simulink model "NCS_Simulation"  (R2019a)
settings: Solver=ode4  StartTime=0.0  StopTime=200  FixedStep=0.004  MaxStep=0.01  RelTol=1e-3
values from neighbouring files (symbols this model uses):
  CAN2EthernetDelay = 0.000    (= 0)    [Parameter.m]
  CycleTime_Sensor = 1/1000    (= 0.001)    [Parameter.m]
  Ethernet2CANDelay = 0.005    [Parameter.m]
  n = 0.001    [Parameter.m]
  nW_ges = 8    [Parameter.m]
  ReferenceDelay = 0.0    (= 0)    [Parameter.m]
undefined symbols (not defined in the file or in its folder): BUSCapacity, controlGate, entity, m, ReadData, ReadSize, v0
libraries: NCS_Library x250, simulink x12
(part 3 of 3)

== system NCS_Simulation/Network/Ethernet (Ring) CAN/Consist 1/Fieldbus 1/Gateway1/CAN Interface/Save Data ==
  Type : Inport
  Data : Inport  Port=2
  FLUSH : Inport  Port=3
  Add : Sum
  Delay : Delay  DelayLength=1  InitialCondition=1
  Detect Change : simulink/Logic and Bit Operations/Detect Change  vinit=0  OutDataTypeStr=boolean
  Detect Change1 : simulink/Logic and Bit Operations/Detect Change  vinit=0  OutDataTypeStr=boolean
  Display : Display
  Display1 : Display
  Display2 : Display
  Hold Data : Stateflow chart  TreatAsAtomicUnit=on
  MATLAB Function : MATLAB Function  TreatAsAtomicUnit=on
  Memory : Memory  InheritSampleTime=on
  OutData : Outport
  wires:
  Hold Data/1(OutData) -> Display/1, OutData/1
  Delay/1 -> MATLAB Function/1(refresh)
  Data/1 -> Detect Change1/1, MATLAB Function/4(Data), Display1/1
  Type/1 -> Detect Change/1, MATLAB Function/3(Type), Display2/1
  MATLAB Function/1(M_Data) -> Memory/1, Hold Data/2(InData)
  FLUSH/1 -> Delay/1, Hold Data/1(Flush)
  Memory/1 -> MATLAB Function/5(M_Data_old)
  Add/1 -> MATLAB Function/2(write)
  Detect Change/1 -> Add/1
  Detect Change1/1 -> Add/2

== system NCS_Simulation/Network/Ethernet (Ring) CAN/Consist 1/Fieldbus 1/Gateway1/Ethernet Interface/Enabled Subsystem ==
  In1 : Inport
  Enable : EnablePort
  Out1 : Outport
  wires:
  In1/1 -> Out1/1

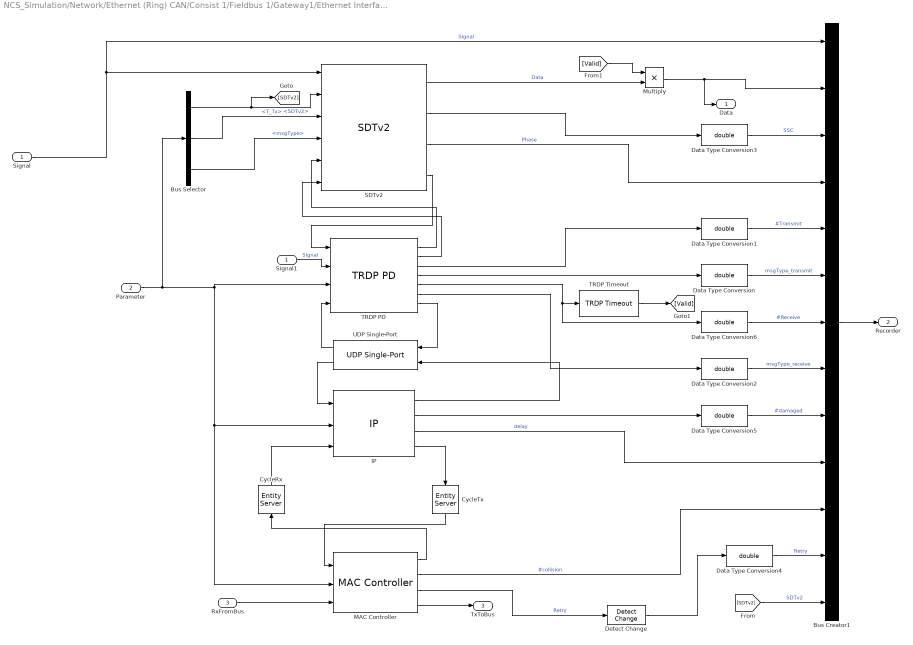
== system NCS_Simulation/Network/Ethernet (Ring) CAN/Consist 1/Fieldbus 1/Gateway1/Ethernet Interface/Protocol Stack ==
  Signal : Inport
  Parameter : Inport  Port=2
  RxFromBus : Inport  Port=3
  Bus Creator1 : BusCreator  Inputs=13
  Bus Selector : BusSelector  OutputSignals=SDTv2,T_Tx,msgType
  CycleRx : EntityServer  InputPortMessageModes=m  OutputPortMessageModes=m  Capacity=inf  ServiceTimeValue=CycleRx
  CycleTx : EntityServer  InputPortMessageModes=m  OutputPortMessageModes=m  Capacity=inf  ServiceTimeValue=CycleTx
  Data Type Conversion{,1..6} (7 alike) : DataTypeConversion  OutDataTypeStr=double
  Detect Change : simulink/Logic and Bit Operations/Detect Change  vinit=0  OutDataTypeStr=boolean
  IP : NCS_Library/Network/ETB/OSI Layers/IP  SystemSampleTime=-1
  MAC Controller : NCS_Library/Network/ETB/OSI Layers/MAC Controller  SystemSampleTime=-1
  Multiply : Product
  SDTv2 : NCS_Library/Network/ETB/OSI Layers/SDTv2  SystemSampleTime=-1
  Signal1 : InportShadow
  TRDP PD : NCS_Library/Network/ETB/OSI Layers/TRDP PD  SystemSampleTime=-1
  TRDP Timeout : NCS_Library/Network/ETB/OSI Layers/TRDP Timeout  SystemSampleTime=-1
  UDP Single-Port : NCS_Library/Network/ETB/OSI Layers/UDP Single-Port  SystemSampleTime=-1
  Data : Outport
  Recorder : Outport  Port=2
  TxToBus : Outport  Port=3
  wires:
  TRDP Timeout/1 -> [Valid]
  [Valid] -> Multiply/1
  SDTv2/1 -> Multiply/2  "Data"
  Multiply/1 -> Bus Creator1/2, Data/1
  Signal1/1 -> TRDP PD/2  "Signal"
  CycleTx/1 -> MAC Controller/1
  IP/4 -> CycleTx/1
  MAC Controller/1 -> CycleRx/1
  CycleRx/1 -> IP/3
  IP/3 -> Bus Creator1/10  "delay"
  IP/2 -> Data Type Conversion5/1
  TRDP PD/6 -> Data Type Conversion2/1
  TRDP PD/5 -> Data Type Conversion6/1, TRDP Timeout/1
  TRDP PD/4 -> Data Type Conversion/1
  TRDP PD/3 -> Data Type Conversion1/1
  SDTv2/3 -> Bus Creator1/4  "Phase"
  SDTv2/2 -> Data Type Conversion3/1
  [SDTv2] -> Bus Creator1/13  "SDTv2"
  RxFromBus/1 -> MAC Controller/3
  UDP Single-Port/2 -> IP/1
  IP/1 -> UDP Single-Port/2
  UDP Single-Port/1 -> TRDP PD/4
  MAC Controller/2 -> Bus Creator1/11  "#collision"
  Signal/1 -> Bus Creator1/1, SDTv2/1  "Signal"
  Parameter/1 -> Bus Selector/1, IP/2, MAC Controller/2, TRDP PD/3
  Data Type Conversion/1 -> Bus Creator1/6  "msgType_transmit"
  Bus Creator1/1 -> Recorder/1
  TRDP PD/7 -> UDP Single-Port/1
  SDTv2/4 -> TRDP PD/1
  TRDP PD/2 -> SDTv2/6
  Bus Selector/2 -> SDTv2/3  "<T_Tx>"
  TRDP PD/1 -> SDTv2/5
  Bus Selector/3 -> SDTv2/4  "<msgType>"
  MAC Controller/4 -> TxToBus/1
  MAC Controller/3 -> Detect Change/1  "Retry"
  Detect Change/1 -> Data Type Conversion4/1
  Bus Selector/1 -> [SDTv2], SDTv2/2  "<SDTv2>"
  Data Type Conversion1/1 -> Bus Creator1/5  "#Transmit"
  Data Type Conversion2/1 -> Bus Creator1/8  "msgType_receive"
  Data Type Conversion3/1 -> Bus Creator1/3  "SSC"
  Data Type Conversion4/1 -> Bus Creator1/12  "Retry"
  Data Type Conversion5/1 -> Bus Creator1/9  "#damaged"
  Data Type Conversion6/1 -> Bus Creator1/7  "#Receive"

== system NCS_Simulation/Network/Ethernet (Ring) CAN/Consist 1/Fieldbus 1/Gateway1/Ethernet Interface/Subsystem4 ==
  Data : Inport
  Add3 : Sum  Inputs=-+-+
  Chart : Stateflow chart  TreatAsAtomicUnit=on
  Clock : Clock
  Compare To Zero1 : simulink/Logic and Bit Operations/Compare To Zero  relop=>=  OutDataTypeStr=uint8
  Constant8 : Constant  Value=T_Tx_CAN
  Constant9 : Constant  Value=1e-10
  Detect Change : simulink/Logic and Bit Operations/Detect Change  vinit=0  OutDataTypeStr=boolean
  Display : Display
  Display1 : Display
  Display2 : Display
  MATLAB Function : MATLAB Function  TreatAsAtomicUnit=on
  Memory1 : Memory  InheritSampleTime=on
  Multiply1 : Product
  Save num release : Subsystem
  Push : Outport
  wires:
  MATLAB Function/1(NEW) -> Display/1, Chart/2(NEW)
  Detect Change/1 -> MATLAB Function/2(Change)
  Compare To Zero1/1 -> Chart/1(TIME), Display1/1, Save num release/Enable
  Chart/1(Push) -> Push/1
  Data/1 -> MATLAB Function/1(Data), Detect Change/1, Display2/1
  Clock/1 -> Add3/2
  Multiply1/1 -> Add3/1
  Memory1/1 -> Multiply1/1, Save num release/1(Time)
  Constant8/1 -> Add3/3, Multiply1/2  "T_Tx"
  Save num release/1(Out1) -> Memory1/1
  Constant9/1 -> Add3/4  "Compensate numeric drift"
  Add3/1 -> Compare To Zero1/1

== system NCS_Simulation/Network/Ethernet (Ring) CAN/Consist 1/Fieldbus 1/Gateway1/Ethernet Interface/User Interface ==
  note: User defined Parameters
  Add : Sum  Inputs=+-
  Bus Creator : BusCreator  Inputs=8
  Constant : Constant  Value=Address  OutDataTypeStr=uint16
  Constant1 : Constant  Value=Destination  OutDataTypeStr=uint16
  Constant2 : Constant  Value=0  OutDataTypeStr=double
  Constant3 : Constant  Value=3  OutDataTypeStr=uint8
  Constant4 : Constant  Value=SDTv2  OutDataTypeStr=double
  Constant5 : Constant
  Constant6 : Constant  Value=Port  OutDataTypeStr=uint16
  Constant7 : Constant  Value=ReplyAddress  OutDataTypeStr=uint16
  MATLAB Function : MATLAB Function  TreatAsAtomicUnit=on
  MATLAB Function1 : MATLAB Function  TreatAsAtomicUnit=on
  Subscribe : Constant  Value=Subscribe  OutDataTypeStr=uint16
  Subsystem1 : Subsystem
  Subsystem2 : Subsystem
  Subsystem3 : Subsystem
  Out1 : Outport
  wires:
  Bus Creator/1 -> Out1/1
  Constant7/1 -> Subsystem3/1(In1)
  Constant5/1 -> Add/2
  Constant2/1 -> Bus Creator/6  "T_Tx"
  Constant1/1 -> Subsystem2/1(In1)
  Subsystem2/1(Out1) -> Bus Creator/2  "Destination"
  MATLAB Function/1(msgType) -> Bus Creator/7  "msgType"
  Subsystem3/1(Out1) -> Bus Creator/4  "ReplyAddress"
  Constant3/1 -> MATLAB Function/1(u)
  Subsystem1/1(Out1) -> Bus Creator/1  "Address"
  Constant/1 -> Subsystem1/1(In1)
  Constant4/1 -> Add/1
  MATLAB Function1/1(y) -> Bus Creator/3  "Subscribe"
  Constant6/1 -> Bus Creator/5  "Port"
  Subscribe/1 -> MATLAB Function1/1(u)
  Add/1 -> Bus Creator/8  "SDTv2"

== system NCS_Simulation/Network/Ethernet (Ring) CAN/Consist 1/Fieldbus 1/Gateway1/CAN Interface/CAN Interface/Re-Transmission Control ==
  IN : Inport
  ReTX : Inport  Port=2
  Reset : Inport  Port=3
  Discard Saved Message upon Success : EntityGate  InputPortMessageModes=m,m  OutputPortMessageModes=m  OperatingMode=Release gate
  Entity Sink : EntityTerminator  InputPortMessageModes=m  NumberEntitiesArrived=on
      settings: OutputPortMap=o0
  Re-Transmission Decision : EntityOutputSwitch  InputPortMessageModes=m  OutputPortMessageModes=m,m  SwitchAttributeName=Attribute1
  Re-transmit Saved Message upon Failure : EntityGate  InputPortMessageModes=m,m  OutputPortMessageModes=m  OperatingMode=Release gate
  OUT : Outport
  #TX : Outport  Port=2
  wires:
  Reset/1 -> Discard Saved Message upon Success/1
  ReTX/1 -> Re-transmit Saved Message upon Failure/1
  Entity Sink/1 -> #TX/1
  Discard Saved Message upon Success/1 -> Entity Sink/1
  Re-Transmission Decision/2 -> Discard Saved Message upon Success/2
  Re-transmit Saved Message upon Failure/1 -> OUT/1
  Re-Transmission Decision/1 -> Re-transmit Saved Message upon Failure/2
  IN/1 -> Re-Transmission Decision/1

== system NCS_Simulation/Network/Ethernet (Ring) CAN/Consist 1/Fieldbus 1/Gateway1/CAN Interface/CAN Interface/Reception Control/Compute ==
  rx_id : Inport  OutDataTypeStr=double  PortDimensions=1
  loss : Inport  Port=2  OutDataTypeStr=double  PortDimensions=1
  rx_rtr : Inport  Port=3  OutDataTypeStr=double  PortDimensions=1
  rx_data : Inport  Port=4  OutDataTypeStr=double  PortDimensions=1
  tx_id : Inport  Port=5  OutDataTypeStr=double  PortDimensions=1
  tx_rtr : Inport  Port=6  OutDataTypeStr=double  PortDimensions=1
  tx_data : Inport  Port=7  OutDataTypeStr=double  PortDimensions=1
  f : TriggerPort  TriggerType=function-call  VariantControl=Variant
      settings: CopyFcn=Stateflow.SLINSF.SimulinkMan.removeBlockPreDeleteFcn  PreDeleteFcn=Stateflow.SLINSF.SimulinkMan.unsafePredeleteFcn
  Lookup Table : Lookup  InputValues=IDRange  Table=2*ones(1,length(IDRange))-IDSubscription  LUTDesignUseExistingBP=off  LUTDesignAbsError=NaN
  MATLAB Function : MATLAB Function  TreatAsAtomicUnit=on
  Sum : Sum  Inputs=|++
  Status : Outport
  Ack : Outport  Port=2
  wires:
  tx_id/1 -> MATLAB Function/4(ID1)
  rx_rtr/1 -> MATLAB Function/2(RTR0)
  rx_id/1 -> MATLAB Function/1(ID0), Lookup Table/1
  Lookup Table/1 -> Sum/1
  loss/1 -> Sum/2, MATLAB Function/7(Loss)
  rx_data/1 -> MATLAB Function/3(Data0)
  tx_data/1 -> MATLAB Function/6(Data1)
  tx_rtr/1 -> MATLAB Function/5(RTR1)
  Sum/1 -> Status/1
  MATLAB Function/1(ACK) -> Ack/1

== system NCS_Simulation/Network/Ethernet (Ring) CAN/Consist 1/Fieldbus 1/Gateway1/CAN Interface/CAN Interface/Signal To CAN Message ==
  Data : Inport
  Entity Generator : EntityGenerator  OutputPortMessageModes=m  Period=T_Tx_CAN  GenerateEntityAtSimulationStart=off  GenerateAction=[entity.ID,entity.RTR,entity.Size,entity.f_St,entity.CommDelay,entity.Time, entity.SensorType] = initMessage();  AttributeName=ID|RTR|Size|Data|CommDelay|RndLoss  AttributeInitialValue=1|1|1|1|1|0  EntityType=Bus object  EntityTypeName=CAN_Message  EntityPriority=MsgID
  Set the Attributes of Messages : Subsystem  TreatAsAtomicUnit=on
  MsgOut : Outport
  wires:
  Data/1 -> Set the Attributes of Messages/1(InData)
  Entity Generator/1 -> MsgOut/1

== system NCS_Simulation/Network/Ethernet (Ring) CAN/Consist 1/Fieldbus 1/Gateway1/CAN Interface/CAN Interface/Simulink Function ==
  controlGate : TriggerPort  TriggerType=function-call  IsSimulinkFunction=on  FunctionName=controlGate  FunctionVisibility=scoped  VariantControl=Variant
  Message Send : MessageSend  OutputPortMessageModes=m
      settings: InputPortMap=u1
  u : ArgIn  DisableCoverage=on  ArgumentName=u
  ctrl : Outport
  wires:
  u/1 -> Message Send/1
  Message Send/1 -> ctrl/1

== system NCS_Simulation/Network/Ethernet (Ring) CAN/Consist 1/Fieldbus 1/Gateway1/CAN Interface/Entry Control/Enabled Subsystem ==
  Enable : EnablePort  StatesWhenEnabling=reset
  Constant : Constant
  Message Send3 : MessageSend  OutputPortMessageModes=m
      settings: InputPortMap=u1
  Out1 : Outport  OutputWhenDisabled=reset  InitialOutput=1
  wires:
  Message Send3/1 -> Out1/1
  Constant/1 -> Message Send3/1

== system NCS_Simulation/Network/Ethernet (Ring) CAN/Consist 1/Fieldbus 1/Gateway1/CAN Interface/Gate Control/Save last release time1 ==
  Time : Inport
  Enable : EnablePort
  Add : Sum
  Constant : Constant  OutDataTypeStr=uint32
  Data Type Conversion : DataTypeConversion  OutDataTypeStr=double
  Display : Display
  Out1 : Outport  InitialOutput=0
  wires:
  Time/1 -> Add/1
  Add/1 -> Data Type Conversion/1
  Constant/1 -> Add/2
  Data Type Conversion/1 -> Display/1, Out1/1

== system NCS_Simulation/Network/Ethernet (Ring) CAN/Consist 1/Fieldbus 1/Gateway1/Ethernet Interface/Subsystem4/Save num release ==
  Time : Inport
  Enable : EnablePort
  Add : Sum
  Constant : Constant  OutDataTypeStr=uint32
  Data Type Conversion : DataTypeConversion  OutDataTypeStr=double
  Display : Display
  Out1 : Outport  InitialOutput=0
  wires:
  Data Type Conversion/1 -> Out1/1, Display/1
  Constant/1 -> Add/2
  Add/1 -> Data Type Conversion/1
  Time/1 -> Add/1

== system NCS_Simulation/Network/Ethernet (Ring) CAN/Consist 1/Fieldbus 1/Gateway1/Ethernet Interface/User Interface/Subsystem1 ==
  In1 : Inport
  Constant : Constant  Value=0  OutDataTypeStr=uint16
  Constant1 : Constant  Value=0  OutDataTypeStr=uint16
  Mux : Mux  Inputs=3
  Out1 : Outport
  wires:
  Constant1/1 -> Mux/3
  Constant/1 -> Mux/2
  Mux/1 -> Out1/1
  In1/1 -> Mux/1

== system NCS_Simulation/Network/Ethernet (Ring) CAN/Consist 1/Fieldbus 1/Gateway1/Ethernet Interface/User Interface/Subsystem2 ==
  In1 : Inport
  Constant : Constant  Value=0  OutDataTypeStr=uint16
  Constant1 : Constant  Value=0  OutDataTypeStr=uint16
  Mux : Mux  Inputs=3
  Out1 : Outport
  wires:
  In1/1 -> Mux/1
  Mux/1 -> Out1/1
  Constant/1 -> Mux/2
  Constant1/1 -> Mux/3

== system NCS_Simulation/Network/Ethernet (Ring) CAN/Consist 1/Fieldbus 1/Gateway1/Ethernet Interface/User Interface/Subsystem3 ==
  In1 : Inport
  Constant : Constant  Value=0  OutDataTypeStr=uint16
  Constant1 : Constant  Value=0  OutDataTypeStr=uint16
  Mux : Mux  Inputs=3
  Out1 : Outport
  wires:
  Constant1/1 -> Mux/3
  Constant/1 -> Mux/2
  Mux/1 -> Out1/1
  In1/1 -> Mux/1

== system NCS_Simulation/Network/Ethernet (Ring) CAN/Consist 1/Fieldbus 1/Gateway1/CAN Interface/CAN Interface/Signal To CAN Message/Set the Attributes of Messages ==
  InData : Inport
  initMessage : TriggerPort  TriggerType=function-call  IsSimulinkFunction=on  FunctionName=initMessage  FunctionVisibility=scoped  VariantControl=Variant
  CommDelay : Constant  Value=(49+8*MsgSize)/BUSCapacity  SampleTime=-1
  Constant : Constant  Value=SensorType  OutDataTypeStr=uint8
  Digital Clock : DigitalClock  SampleTime=-1
  ID : Constant  Value=MsgID  SampleTime=-1
  RTR : Constant  Value=0  SampleTime=-1
  Size : Constant  Value=MsgSize  SampleTime=-1
  ID~ : ArgOut  ArgumentName=ID
  RTR~ : ArgOut  Port=2  ArgumentName=RTR
  Size~ : ArgOut  Port=3  ArgumentName=Size
  Data : ArgOut  Port=4  PortDimensions=[3 1]  ArgumentName=Data
  CommDelay~ : ArgOut  Port=5  ArgumentName=CommDelay
  Time : ArgOut  Port=6  ArgumentName=Time
  Type : ArgOut  Port=7  OutDataTypeStr=uint8  ArgumentName=Type
  wires:
  Constant/1 -> Type/1
  Digital Clock/1 -> Time/1
  Size/1 -> Size~/1
  RTR/1 -> RTR~/1
  ID/1 -> ID~/1
  CommDelay/1 -> CommDelay~/1
  InData/1 -> Data/1

== matlab function NCS_Simulation/Network/Ethernet (Ring) CAN/Consist 2/Output Control/MATLAB Function ==
  data: in_Y_M input; in_U input; out output
function out = Mux(in_Y_M,in_U)

out = [ in_Y_M, in_U ];

== matlab function NCS_Simulation/Network/Ethernet (Ring) CAN/Consist 1/Fieldbus 1/Gateway1/Ethernet Interface/MATLAB Function ==
  data: u input; y output
function y = fcn(u)

y = u(:,2);

== matlab function NCS_Simulation/Network/Ethernet (Line) CAN/Consist 2/Output Control/MATLAB Function ==
  data: in_Y_M input; in_U input; out output
function out = Mux(in_Y_M,in_U)

out = [ in_Y_M, in_U ];

== stateflow chart NCS_Simulation/Network/Ethernet (Ring) CAN/Consist 1/Fieldbus 1/Gateway1/CAN Interface/CAN Interface/Reception Control ==
  settings: enableNonTerminalStates=1
  state Process
    en:
    Port.data=S;
    send(Port);
  state [Status,Ack] = Compute(rx_id,loss,rx_rtr,rx_data,tx_id,tx_rtr,tx_data) [function]
  (default) -> Process : {S=1; Ack=0; TX_ID=-1; TX_RTR=0; TX_Data=0;}
  Process -> Process [order 1] : TX{TX_ID=TX.data.ID; TX_RTR=TX.data.RTR; TX_Data=TX.data.Data;}
  (junction 12) -> Process [order 1] : [Ack==1]{Success.data=1; send(Success);}
  (junction 12) -> Process [order 2] : [Ack==0]{ReTX.data=1; send(ReTX);}
  Process -> (junction 12) [order 2] : RX{[S,Ack]=Compute(RX.data.ID,...
      |                         RX.data.RndLoss, ...
      |                         RX.data.RTR, ...
      |                         RX.data.Data, ...
      |                         TX_ID, ...
      |                         TX_RTR, ...
      |                         TX_Data);}
  data: Status function_output; Ack function_output; rx_id function_input double size=1; loss function_input double size=1; rx_rtr function_input double size=1; rx_data function_input double size=1; tx_id function_input double size=1; tx_rtr function_input double size=1; tx_data function_input double size=1; TX input Bus: CAN_Message; RX input Bus: CAN_Message; S local; Ack local; TX_ID local; TX_RTR local; TX_Data local; Port output; Success output; ReTX output

== matlab function NCS_Simulation/Network/Ethernet (Ring) CAN/Consist 1/Fieldbus 1/Gateway1/CAN Interface/CAN Interface/Reception Control/Compute/MATLAB Function ==
  data: ID0 input; ACK output; RTR0 input; Data0 input; ID1 input; RTR1 input; Data1 input; Loss input
function ACK = fcn(ID0,RTR0,Data0,ID1,RTR1,Data1,Loss)
% Compare the message ID, RTR, Data fields to acknowledge a successful send

if (ID0 == ID1 && RTR0 == RTR1 && Data0 == Data1 && Loss < 1)
    ACK = 1;
else
    ACK = 0;
end

== stateflow chart NCS_Simulation/Network/Ethernet (Ring) CAN/Consist 1/Fieldbus 1/Gateway1/CAN Interface/Save Data/Hold Data ==
  state Init
    en: SavedData=InData;
  state Save_Data
    du: OutData=SavedData;
  state Push_Data
    en: OutData=SavedData;
  (default) -> Init
  Init -> Save_Data
  Push_Data -> Save_Data
  Save_Data -> Push_Data : [Flush==1]{SavedData=InData;}
  data: Flush input; InData input; SavedData local; OutData output

== matlab function NCS_Simulation/Network/Ethernet (Ring) CAN/Consist 1/Fieldbus 1/Gateway1/CAN Interface/Save Data/MATLAB Function ==
  data: refresh input; write input; Type input; Data input; M_Data output; M_Data_old input
function M_Data = SaveData (refresh, write, Type, Data, M_Data_old)
%% Init
M_Data = zeros(3,20);
M_Data(1,1) = 1;

if refresh
    % refresh matrix
else
    % save data in matrix
    M_Data = M_Data_old;
    if write && Type > 0 && Type < 3
        if M_Data(1,1) == 1
            % no data saved yet
            M_Data(Type,2) = Data;          % save data
            M_Data(1,1) = M_Data(1,1)+1;    % update length
        else
            % compare the data to write with the data already saved in the matrix
            for i=2:M_Data(1,1)+1
                if M_Data(1,i) ~= 0 || M_Data(2,i) ~= 0 || M_Data(3,i) ~= 0
                    % there is data at current position
                    if M_Data(Type,i) == Data
                        % data on current position is data to write
                        break;  % data already saved in Ethernet entity
                    end
                else
                    M_Data(Type,i) = Data;          % save data
                    M_Data(1,1) = M_Data(1,1)+1;    % update length
                    break;  % finished
                end
            end % endfor
        end
    end %endif write
end % endif refresh
end % function

== matlab function NCS_Simulation/Network/Ethernet (Ring) CAN/Consist 2/ED/User Interface/MATLAB Function ==
  data: u input; msgType output
function msgType = GetmsgType(u)

switch u
    case 1
        msgType = 11;
    case 2
        msgType = 13;
    case 3
        msgType = 13;
    otherwise
        msgType = 0;
end
end % end function

== matlab function NCS_Simulation/Network/Ethernet (Ring) CAN/Consist 1/Fieldbus 1/Gateway1/Ethernet Interface/Buffer ==
  data: updatedBuffer input; Push input; Buffer output; Data input; data output
function [Buffer, data] = GatewayBuffer(updatedBuffer, Push, Data)

%% Init
Buffer = zeros(3,100);
FIN = 0;

Buffer = updatedBuffer;
%% Write to buffer
for i=2:Data(1,1)
    for j=1:length(Buffer)
        if Buffer(1,j) == 0 && Buffer(2,j) == 0 && Buffer(3,j) == 0
            % free position
            % save data
            Buffer(:,j) = Data(:,i);
            break;

        elseif Data(1,i) == Buffer(1,j) && Data(2,i) == Buffer(2,j) && Data(3,i) == Buffer(3,j)
            % data already in buffer
            FIN = 1;
            break;
        end
    end % end for
    
    if FIN
        % data already in buffer
        break;
    end
end % end for

%% Push
if Push
    % Read from buffer
    data = Buffer(:,1);

    % Udpdate buffer
    Buffer(:,1:length(Buffer)-1) = Buffer(:,2:length(Buffer));
else
    data = [0;0;0];
end

end % end function

== matlab function NCS_Simulation/Network/Ethernet (Ring) CAN/Consist 1/Fieldbus 1/Gateway1/Ethernet Interface/User Interface/MATLAB Function ==
  data: u input; msgType output
function msgType = GetmsgType(u)

switch u
    case 1
        msgType = 11;
    case 2
        msgType = 13;
    case 3
        msgType = 13;
    otherwise
        msgType = 0;
end
end % end function

== matlab function NCS_Simulation/Network/Ethernet (Ring) CAN/Consist 1/Fieldbus 1/Gateway1/Ethernet Interface/User Interface/MATLAB Function1 ==
  data: u input; y output
function y = fcn(u)

m = length(u);
ADD = zeros(m,2);
y = [u ADD];

== matlab function NCS_Simulation/Network/Ethernet (Ring) CAN/Consist 2/ED/User Interface/MATLAB Function1 ==
  data: u input; y output
function y = fcn(u)

m = length(u);
ADD = zeros(m,2);
y = [u ADD];

== matlab function NCS_Simulation/Network/Ethernet (Ring) CAN/Consist 2/ED/User Interface/Subsystem2/MATLAB Function ==
  data: u input; y output
function y = fcn(u)

y = uint16( zeros(4,1) );
y(1) = u(1);
y(2) = u(2);

== matlab function NCS_Simulation/Network/Ethernet (Ring) CAN/Consist 1/Fieldbus 1/Gateway1/Ethernet Interface/Subsystem4/MATLAB Function ==
  data: Data input; NEW output; Change input
function NEW = DetectNewData(Data, Change)

NEW = 0;
changed = 0;
for i=1:3
    for j=1:20
        if Change(i,j) ~= 0
            changed = 1;
            break;
        end
    end
end
        
if changed
    if Data(1,1) < 2
        % Data is empty
        NEW = 0;
    else
        % New Data
        NEW = Data(1,1)-1;
    end
end

end

== stateflow chart NCS_Simulation/Network/Ethernet (Ring) CAN/Consist 1/Fieldbus 1/Gateway1/Ethernet Interface/Subsystem4/Chart ==
  state Buffer_empty
    en: n=0;
    en: Push = 0;
  state Buffer_full
    du: Push=0;
  (default) -> Buffer_empty
  Buffer_full -> Buffer_empty [order 4] : [n==0]
  Buffer_empty -> Buffer_full [order 1] : [NEW>0]{n=n+NEW;}
  Buffer_empty -> Buffer_full [order 2] : [n>0]
  Buffer_full -> Buffer_full [order 1] : [NEW>0&&TIME==1]{n=n+NEW-1;}
  Buffer_full -> Buffer_full [order 3] : [TIME==1]{n=n-1;Push=1;}
  Buffer_full -> Buffer_full [order 2] : [NEW>0]{n=n+NEW}
  data: TIME input; n local; NEW input; Push output
